simulink model "super_eplus_cases"  (R2014a)
settings: Solver=ode3  StartTime=0.0  StopTime=24*3600  FixedStep=300  RelTol=1e-3
libraries: refrigeration x1
settings Model: Creator=avenger  LastModifiedBy=avenger
settings DataIOCC: LimitDataPoints=off

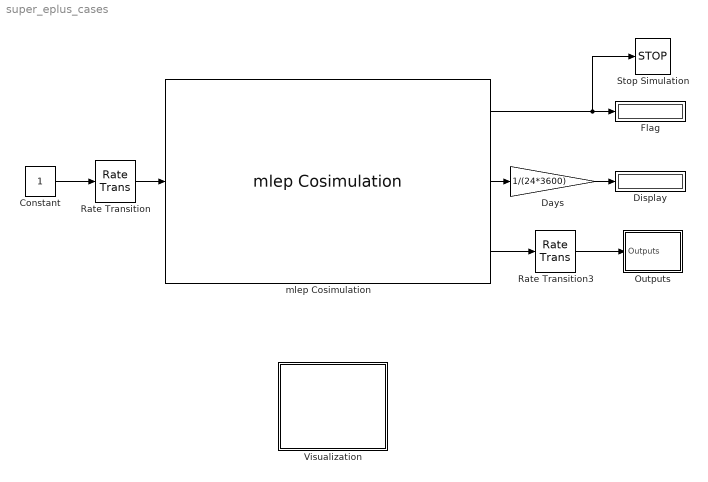
== system super_eplus_cases ==
  Constant : Constant
  Days : Gain  Gain=1/(24*3600)
  Display : Display
  Flag : Display
  Outputs : Subsystem
  Rate Transition : RateTransition
  Rate Transition3 : RateTransition
  Stop Simulation : Stop
  Visualization : Subsystem
  mlep Cosimulation : refrigeration/mlep Cosimulation  progname='runenergyplus'  idf='super_noSizing'  weather='USA_FL_Miami.Intl.AP.722020_TMY3'  timeout=2000  step=300  numinput=1  numoutput=21  bcvtbpath='/home/avenger/Documents/git/mlep_v2.0/MLE+/bcvtb'
  wires:
  mlep Cosimulation/2 -> Days/1
  mlep Cosimulation/1 -> Stop Simulation/1, Flag/1
  mlep Cosimulation/3 -> Rate Transition3/1
  Days/1 -> Display/1
  Rate Transition3/1 -> Outputs/1(Outputs)
  Constant/1 -> Rate Transition/1
  Rate Transition/1 -> mlep Cosimulation/1

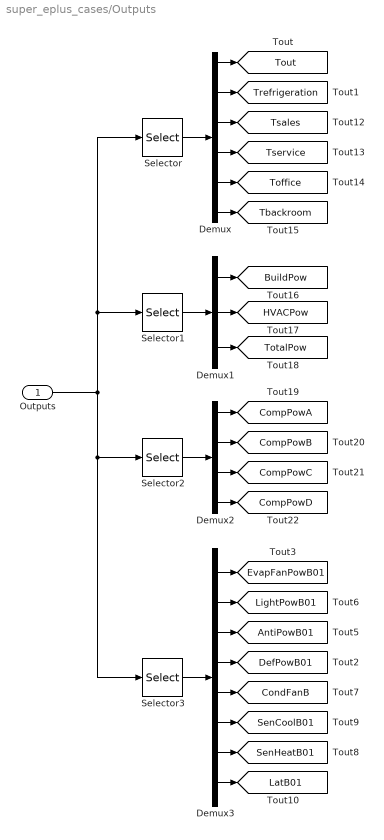
== system super_eplus_cases/Outputs ==
  Outputs : Inport
  Demux : Demux  Outputs=6
  Demux1 : Demux  Outputs=3
  Demux2 : Demux
  Demux3 : Demux  Outputs=8
  Selector : Selector  InputPortWidth=21  Indices=[1:6]
  Selector1 : Selector  InputPortWidth=21  Indices=[7:9]
  Selector2 : Selector  InputPortWidth=21  Indices=[10:13]
  Selector3 : Selector  InputPortWidth=21  Indices=[14:21]
  tag scope: AntiPowB01=global, BuildPow=global, CompPowA=global, CompPowB=global, CompPowC=global, CompPowD=global, CondFanB=global, DefPowB01=global, EvapFanPowB01=global, HVACPow=global, LatB01=global, LightPowB01=global, SenCoolB01=global, SenHeatB01=global, Tbackroom=global, Toffice=global, TotalPow=global, Tout=global, Trefrigeration=global, Tsales=global, Tservice=global
  wires:
  Demux/1 -> [Tout]
  Demux/2 -> [Trefrigeration]
  Demux/3 -> [Tsales]
  Demux/4 -> [Tservice]
  Demux/5 -> [Toffice]
  Demux/6 -> [Tbackroom]
  Selector/1 -> Demux/1
  Selector1/1 -> Demux1/1
  Demux1/1 -> [BuildPow]
  Demux1/2 -> [HVACPow]
  Demux1/3 -> [TotalPow]
  Selector2/1 -> Demux2/1
  Demux2/1 -> [CompPowA]
  Demux2/2 -> [CompPowB]
  Demux2/3 -> [CompPowC]
  Demux2/4 -> [CompPowD]
  Outputs/1 -> Selector/1, Selector1/1, Selector3/1, Selector2/1
  Selector3/1 -> Demux3/1
  Demux3/1 -> [EvapFanPowB01]
  Demux3/2 -> [LightPowB01]
  Demux3/3 -> [AntiPowB01]
  Demux3/4 -> [DefPowB01]
  Demux3/5 -> [CondFanB]
  Demux3/6 -> [SenCoolB01]
  Demux3/7 -> [SenHeatB01]
  Demux3/8 -> [LatB01]

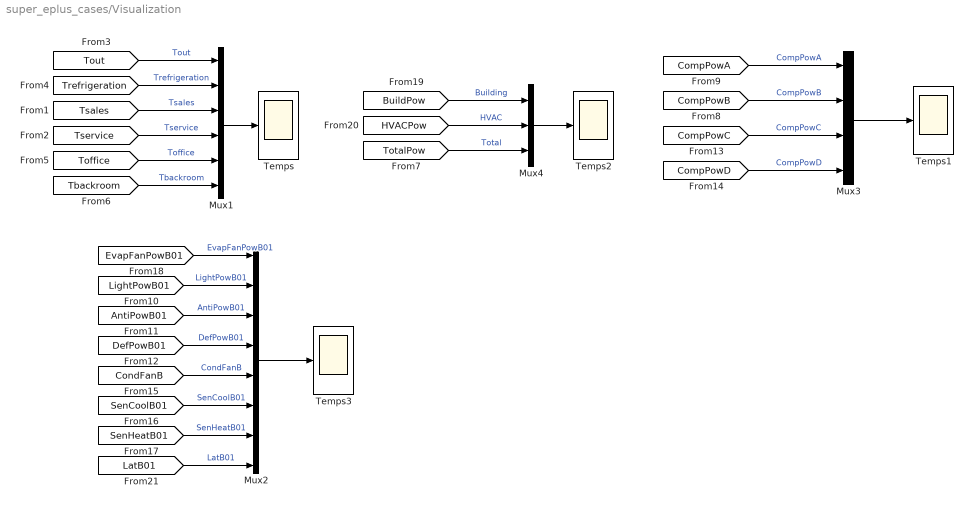
== system super_eplus_cases/Visualization ==
  Mux1 : Mux  Inputs=6
  Mux2 : Mux  Inputs=8
  Mux3 : Mux
  Mux4 : Mux  Inputs=3
  Temps{,1..3} (4 alike) : Scope
      Temps settings: ShowLegends=on  TimeRange=90000  YMin=10  YMax=35
      Temps1 settings: ShowLegends=on  TimeRange=90000  YMin=0  YMax=35000
      Temps2 settings: ShowLegends=on  TimeRange=90000  YMin=0  YMax=600000  SaveName=ScopeData2
      Temps3 settings: ShowLegends=on  TimeRange=90000  YMin=-2000  YMax=14000  SaveName=ScopeData3
  wires:
  Mux1/1 -> Temps/1
  [Tout] -> Mux1/1  "Tout"
  [Trefrigeration] -> Mux1/2  "Trefrigeration"
  [Tsales] -> Mux1/3  "Tsales"
  [Tservice] -> Mux1/4  "Tservice"
  [Toffice] -> Mux1/5  "Toffice"
  [Tbackroom] -> Mux1/6  "Tbackroom"
  [CompPowA] -> Mux3/1  "CompPowA"
  [EvapFanPowB01] -> Mux2/1  "EvapFanPowB01"
  [LightPowB01] -> Mux2/2  "LightPowB01"
  [AntiPowB01] -> Mux2/3  "AntiPowB01"
  Mux4/1 -> Temps2/1
  [HVACPow] -> Mux4/2  "HVAC"
  [TotalPow] -> Mux4/3  "Total"
  [BuildPow] -> Mux4/1  "Building"
  [CompPowB] -> Mux3/2  "CompPowB"
  [CompPowC] -> Mux3/3  "CompPowC"
  [CompPowD] -> Mux3/4  "CompPowD"
  Mux3/1 -> Temps1/1
  [DefPowB01] -> Mux2/4  "DefPowB01"
  [CondFanB] -> Mux2/5  "CondFanB"
  [SenCoolB01] -> Mux2/6  "SenCoolB01"
  [SenHeatB01] -> Mux2/7  "SenHeatB01"
  [LatB01] -> Mux2/8  "LatB01"
  Mux2/1 -> Temps3/1
